simulink model "Notfalltests"  (R2021a)
settings: Solver=VariableStepAuto  StartTime=0.0  StopTime=1  RelTol=1e-3
model workspace (MAT data in the model file):
  Kz = Simulink.Parameter
  Kz.Value = Simulink.data.Expression
  Kz.Value.ExpressionString = "(L/(Lc+ds))"
  Kz.DataType = 'auto'
  Kz.Dimensions = -1
  L = Simulink.Parameter
  L.Value = 52.8
  L.DataType = 'auto'
  L.Dimensions = [1 1]
  Lc = Simulink.Parameter
  Lc.Value = 4.4
  Lc.DataType = 'auto'
  Lc.Dimensions = [1 1]
  Rk = Simulink.Parameter
  Rk.Value = Simulink.data.Expression
  Rk.Value.ExpressionString = "Lc/v"
  Rk.DataType = 'auto'
  Rk.Dimensions = -1
  Tz = Simulink.Parameter
  Tz.Value = Simulink.data.Expression
  Tz.Value.ExpressionString = "L/v"
  Tz.DataType = 'auto'
  Tz.Dimensions = -1
  ds = Simulink.Parameter
  ds.Value = Simulink.data.Expression
  ds.Value.ExpressionString = "dt*v"
  ds.DataType = 'auto'
  ds.Dimensions = -1
  dt = Simulink.Parameter
  dt.Value = 1
  dt.DataType = 'auto'
  dt.Dimensions = [1 1]
  v = Simulink.Parameter
  v.Value = 13.89
  v.DataType = 'auto'
  v.Dimensions = [1 1]
libraries: EdgesLibrary x8, StreetLanesLibrary x6, SourcesAndSinksLibrary x4, simulink x2
settings Model: OrderedModelArguments=off  Creator=phill  LastModifiedBy=phill
settings SolverCC: ZeroCrossAlgorithm=Adaptive

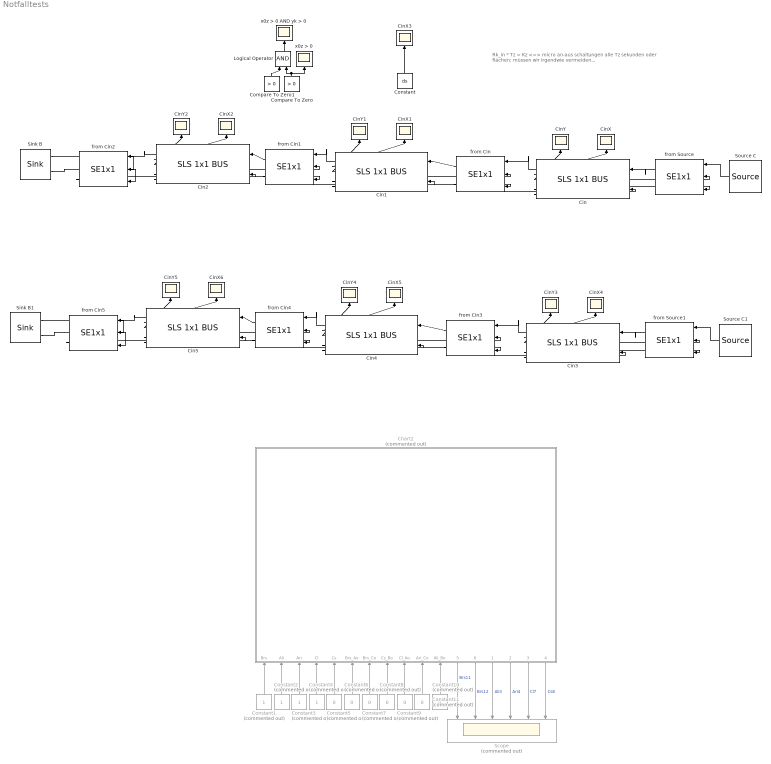
== system Notfalltests ==
  note: Rk_in * Tz = Kz   <=> micro an-aus schaltungen alle Tz sekunden
      | oder flächen; müssen wir irgendwie vermeiden...
  Chart2 : Stateflow chart  Commented=on  TreatAsAtomicUnit=on
      settings: PortSchema="{\"entries\":[{\"content\":{\"sides\":[{\"content\":{\"connectorIds\":[]},\"type\":\"ConnectorPlacement.EquallySpacedRectSide\",\"uuid\":\"dee1a780-e9dd-4205-adb9-3e9cb1ec0cd6\"},{\"content\":{\"connectorIds\":[],\"side\":\"RIGHT\"},\"type\":\"ConnectorPlacement.EquallySpacedRectSide\",\"uuid\":\"bc6af08d-2df8-4a74-93d0-032b7c1c381c\"},{\"content\":{\"connectorIds\":[],\"side\":\"TOP\"},\"type\":\"ConnectorPlacement.EquallySpacedRectSide\",\"uuid\":\"98fea325-c9fc-472d-8e1a-d846d6e99e12\"},{\"content\":{\"connectorIds\":[\"In5\",\"In1\",\"In2\",\"In3\",\"In4\",\"In11\",\"In10\",\"In9\",\"In8\",\"In7\",\"In6\",\"Out5\",\"Out6\",\"Out1\",\"Out2\",\"Out3\",\"Out4\"],\"side\":\"BOTTOM\"},\"type\":\"ConnectorPlacement.EquallySpacedRectSide\",\"uuid\":\"a092283f-ef46-48e2-a5f8-8210ac00b2f9\"}]},\"type\":\"ConnectorPlacement.EquallySpacedConnector\",\"uuid\":\"33a851aa-4180-41c0-b4bb-9b9c3be41936\"}],\"packageUris\":[\"http://schema.mathworks.com/mf0/Connector/R2020b\"],\"version\":\"1.0\"}"
  Cin : StreetLanesLibrary/SLS 1x1 BUS  Kz=2.886  Tz=3.8
  Cin1 : StreetLanesLibrary/SLS 1x1 BUS  Kz=2.886  Tz=3.8
  Cin2 : StreetLanesLibrary/SLS 1x1 BUS  Kz=2.886  Tz=3.8
  Cin3 : StreetLanesLibrary/SLS 1x1 BUS  Kz=1  Tz=1
  Cin4 : StreetLanesLibrary/SLS 1x1 BUS  Kz=1  Tz=1
  Cin5 : StreetLanesLibrary/SLS 1x1 BUS  Kz=1  Tz=1
  CinX{,1..6} (7 alike) : Scope
  CinY{,1..5} (6 alike) : Scope
  Compare To Zero : simulink/Logic and Bit Operations/Compare To Zero  relop=>  OutDataTypeStr=boolean
  Compare To Zero1 : simulink/Logic and Bit Operations/Compare To Zero  relop=>  OutDataTypeStr=boolean
  Constant : Constant  Value=ds
  Constant{1..4} (4 alike) : Constant  Commented=on
  Constant{5..11} (7 alike) : Constant  Commented=on  Value=0
  Logical Operator : Logic  AllPortsSameDT=off  OutDataTypeStr=boolean
  Scope : Scope  Commented=on  NumInputPorts=6
  Sink B : SourcesAndSinksLibrary/Sink  SystemSampleTime=-1  VariantActivationTime=update diagram  Latency=0  AutoFrameSizeCalculation=off
      settings: PortSchema="{\"entries\":[{\"content\":{\"sides\":[{\"content\":{\"connectorIds\":[\"Out1\",\"Out2\"]},\"type\":\"ConnectorPlacement.EquallySpacedRectSide\",\"uuid\":\"9fd2383e-3590-4f0f-bafc-5a4adfbb32b4\"},{\"content\":{\"connectorIds\":[],\"side\":\"RIGHT\"},\"type\":\"ConnectorPlacement.EquallySpacedRectSide\",\"uuid\":\"1e687aa9-1098-45bd-a1f6-ea403f3f2897\"},{\"content\":{\"connectorIds\":[],\"side\":\"TOP\"},\"type\":\"ConnectorPlacement.EquallySpacedRectSide\",\"uuid\":\"fe6eaa71-085c-414b-983a-a0e72e52a49c\"}]},\"type\":\"ConnectorPlacement.EquallySpacedConnector\",\"uuid\":\"370c1712-4373-4726-99c2-6cb04807ece1\"}],\"packageUris\":[\"http://schema.mathworks.com/mf0/Connector/R2020b\"],\"version\":\"1.0\"}"
  Sink B1 : SourcesAndSinksLibrary/Sink  SystemSampleTime=-1  VariantActivationTime=update diagram  Latency=0  AutoFrameSizeCalculation=off
      settings: PortSchema="{\"entries\":[{\"content\":{\"sides\":[{\"content\":{\"connectorIds\":[\"Out1\",\"Out2\"]},\"type\":\"ConnectorPlacement.EquallySpacedRectSide\",\"uuid\":\"9fd2383e-3590-4f0f-bafc-5a4adfbb32b4\"},{\"content\":{\"connectorIds\":[],\"side\":\"RIGHT\"},\"type\":\"ConnectorPlacement.EquallySpacedRectSide\",\"uuid\":\"1e687aa9-1098-45bd-a1f6-ea403f3f2897\"},{\"content\":{\"connectorIds\":[],\"side\":\"TOP\"},\"type\":\"ConnectorPlacement.EquallySpacedRectSide\",\"uuid\":\"fe6eaa71-085c-414b-983a-a0e72e52a49c\"}]},\"type\":\"ConnectorPlacement.EquallySpacedConnector\",\"uuid\":\"370c1712-4373-4726-99c2-6cb04807ece1\"}],\"packageUris\":[\"http://schema.mathworks.com/mf0/Connector/R2020b\"],\"version\":\"1.0\"}"
  Source C : SourcesAndSinksLibrary/Source  SystemSampleTime=-1  VariantActivationTime=update diagram  Latency=0  AutoFrameSizeCalculation=off
  Source C1 : SourcesAndSinksLibrary/Source  SystemSampleTime=-1  VariantActivationTime=update diagram  Latency=0  AutoFrameSizeCalculation=off
  from Cin : EdgesLibrary/SE1x1  Rk=0.32
  from Cin1 : EdgesLibrary/SE1x1  Rk=0.32
  from Cin2 : EdgesLibrary/SE1x1  Rk=0.32
  from Cin3 : EdgesLibrary/SE1x1  Rk=1
  from Cin4 : EdgesLibrary/SE1x1  Rk=1
  from Cin5 : EdgesLibrary/SE1x1  Rk=1
  from Source : EdgesLibrary/SE1x1  Rk=0.32
  from Source1 : EdgesLibrary/SE1x1  Rk=1
  x0z > 0 : Scope
  x0z > 0 AND yk > 0 : Scope
  wires:
  Cin/3 -> CinX/1
  Cin/7 -> from Source/3
  Cin/4 -> CinY/1
  Source C/1 -> from Source/1
  Cin/6 -> from Source/2
  from Source/1 -> Cin/1
  from Cin/2 -> Cin/2
  Cin/2 -> from Cin/1
  Cin1/6 -> from Cin/2
  Cin1/7 -> from Cin/3
  from Cin/1 -> Cin1/1
  Cin1/4 -> CinY1/1
  Cin1/3 -> CinX1/1
  Cin1/2 -> from Cin1/1
  from Cin1/2 -> Cin1/2
  Compare To Zero1/1 -> Logical Operator/1
  Compare To Zero/1 -> Logical Operator/2, x0z > 0/1
  Logical Operator/1 -> x0z > 0 AND yk > 0/1
  Sink B/1 -> from Cin2/2
  Sink B/2 -> from Cin2/3
  Cin2/2 -> from Cin2/1
  from Cin2/2 -> Cin2/2
  Cin2/6 -> from Cin1/2
  Cin2/7 -> from Cin1/3
  from Cin1/1 -> Cin2/1
  Cin2/4 -> CinY2/1
  Cin2/3 -> CinX2/1
  Constant/1 -> CinX3/1
  Constant11/1 -> Chart2/7(Ari_Co)
  Constant9/1 -> Chart2/8(Cl_Ao)
  Constant7/1 -> Chart2/10(Brs_Co)
  Constant3/1 -> Chart2/2(Ari)
  Constant2/1 -> Chart2/1(Ali)
  Constant8/1 -> Chart2/9(Cs_Bo)
  Constant6/1 -> Chart2/11(Brs_Ao)
  Constant1/1 -> Chart2/5(Brs)
  Chart2/6(enableBrs12) -> Scope/2  "Brs12"
  Chart2/1(enableAli3) -> Scope/3  "Ali3"
  Chart2/2(enableAri4) -> Scope/4  "Ari4"
  Constant4/1 -> Chart2/3(Cl)
  Constant10/1 -> Chart2/6(Ali_Bo)
  Chart2/3(enableCl7) -> Scope/5  "Cl7"
  Chart2/4(enableCs8) -> Scope/6  "Cs8"
  Constant5/1 -> Chart2/4(Cs)
  Chart2/5(enableBrs11) -> Scope/1  "Brs11"
  Sink B1/1 -> from Cin5/2
  from Cin4/1 -> Cin5/1
  from Source1/1 -> Cin3/1
  Cin5/7 -> from Cin4/3
  Cin3/6 -> from Source1/2
  from Cin5/2 -> Cin5/2
  Cin5/6 -> from Cin4/2
  Cin5/4 -> CinY5/1
  Cin5/3 -> CinX6/1
  Cin5/2 -> from Cin5/1
  Source C1/1 -> from Source1/1
  Cin4/2 -> from Cin4/1
  Sink B1/2 -> from Cin5/3
  Cin4/7 -> from Cin3/3
  Cin3/2 -> from Cin3/1
  from Cin3/1 -> Cin4/1
  from Cin3/2 -> Cin3/2
  Cin4/6 -> from Cin3/2
  Cin4/4 -> CinY4/1
  Cin3/7 -> from Source1/3
  from Cin4/2 -> Cin4/2
  Cin3/3 -> CinX4/1
  Cin3/4 -> CinY3/1
  Cin4/3 -> CinX5/1

== stateflow chart Notfalltests/Chart2 ==
  note: Notizen (mal auf Deutsch):
      | wenn an einer kante etwas anliegt und keine der stärkeren kanten etwas anliegen hat,
      | und die konfliktbereiche frei sind: schalte kante frei
      | <Ali 3> wird dominiert von <Cl 7> und <Cs 8> [Kreuzungen: <Brs Co> <Cl Ao> <Cs Bo>
      | <Ari 4> wird nicht dominiert [Kreuzungen: <Brs Co>
      | <Cl 7> wird dominiert von <Brs 11> und <Brs 12> [Kreuzungen: <Brs Co> <Brs Ao><Ali Bo>
      | <Cs 8> wird nicht dominiert [Kreuzungen: <Ali Bo>
      | <Brs 11> wird dominiert von <Ali 3> und <Ari 4> [Kreuzungen: <Brs Ao> <Ali Bo> <Ari Co>*<Cl Ao>
      | <Brs 12> wird nicht dominiert [Kreuzungen: <Cl Ao>
      |
      | Anmerkung: die einflüsse Brs11 und Brs12 behindern sich nicht. da beide kanten an
      | EIN UND DEMSELBEN SEGMENT liegen, und unsere 0.5:0.5 gewichtung schon suggeriert,
      | dass sich hier die autos "spalten", können sich die autos beim "Parallelen" fließen
      | in die segmente <Brs Co> und <Brs Ao> nicht wirklich in die quere kommen. Oder selbst wenn sie es
      | tun, können wir nichts dagegen unternehmen - wenn wir einem der pfade gegenüber dem anderen
      | priorität geben, wird bei dem anderen jeweils NIE etwas fließen. Damit müssen wir wohl leben :(
      |
      | a)
      | if [Ali > 0 && Cl == 0 && Cs == 0 && Brs_Co == 0 && Cl_Ao == 0 && Cs_Bo == 0]{enableAli3=1;}
      | else {enableAli3=0;}
      | b)
      | if [Ari > 0 && Brs_Co == 0]{enableAri4=1;}
      | else {enableAri4=0;}
      | c)
      | if [Cl > 0 && Brs == 0 && Brs_Co == 0 && Brs_Ao == 0 && Ali_Bo == 0]{enableCl7=1;}
      | else {enableCl7=0;}
      | d)
      | if [Cs > 0 && Ali_Bo == 0]{enableCs8=1;}
      | else {enableCs8=0;}
      | e)
      | if [Brs > 0 && Ali == 0 && Ari == 0 && Ali_Bo == 0 && Ari_Co == 0 && Cl_Ao]{enableBrs11=1;}
      | else {enableBrs11=0;}
      | f)
      | if [Brs > 0 && Cl_Ao == 0]{enableBrs12=1;}
      | else {enableBrs12=0;}
      |
      | Anmerkung: Da es im Falle [Ali > 0 && Brs > 0 && Cl > 0] einen deadlock gibt, müssen wir uns entscheiden, wer fahren darf.
      |
      | // Brs11 soll das fahrtrecht bekommen, um den fluss entlang der geraden aufrechtzuerhalten, wenn möglich
      | if [Ari == 0 && (Ali_Bo == 0 && Ari_Co == 0 && Cl_Ao == 0)]{enableBrs11=1;}
      | else
      |
      | // falls Brs12 nicht kann, versucht Ali zu fahren. Eigentlich müsste Cl die nächstbeste Wahl sein,
      | // allerdings kann Cl im falle eines Deadlocks ohnehin nicht fließen, da wegen unserer modellierung
      | // der 1x2 kanten (bzw. 1x2 segmente) gilt "Deadlock => [Brs > 0] => [Brs12 will aktiv sein]" - und da
      | // Brs12 vorrang vor Cl7 hat, ist Cl7 in diesem szenario grundsätzlich blockiert.
      | if [Cs == 0 && (Brs_Co == 0 && Cl_Ao == 0 && Cs_Bo == 0)]{enableAli3=1;}
      | else //guess noone can make it
  note: ?
  note: Brs-11-<Brs Co>-6-Co
      | (Links will geradeaus)
  note: Brs-12-<Brs Ao>-1-Ao
      | (Links will geradeaus)
  note: Ari-4-<Ari Co>-5-Co
      | (Unten will rechts abbiegen)
  note: Cl-7-<Cl Ao>-2-Ao
      | (Rechts will links abbiegen)
  note: Cs-8-<Cl Ao>-9-Bo
      | (Rechts will geradeaus)
  note: Ali-3-<Ali Bo>-10-Bo
      | (Unten will Links abbiegen)
  note: Deadlock-Detection
  note: Anstelle der ebene für deadlock resolution konnte man den "Links will geradeaus" bereich in der reihenfolge VOR "Unten will links abbiegen" setzen. "Links will geradeaus" muss dann um eine weitere kante mit höchster priorität ergänzt werden mit einem label
      | [ (Ali > 0 && Brs > 0 && Cl > 0 ) && (Ari == 0 && Ali_Bo == 0 && Ari_Co == 0]{enableBrs11=1;}
      |
      | "Unten will links abbiegen" wird dann ebenfalls um eine Kante mit höchster priorität ergänzt mit dem Label
      | [ (Ali > 0 && Brs > 0 && Cl > 0) && (Cs_Bo == 0 && Cl_Ao == 0) && ~(enableBrs11==1)
  note: Deadlock-Resolution
  (junction 23) -> (junction 29) [order 1] : [Ari > 0 && Brs_Co == 0]{enableAri4=1;}
  (junction 29) -> (junction 36) [order 1] : [Cl > 0 && Brs == 0 && Brs_Co == 0 && Brs_Ao == 0 && Ali_Bo == 0]{enableCl7=1; }
  (junction 39) -> (junction 40) [order 1] : [Brs > 0 && Ali == 0 && Ari == 0 && Ali_Bo == 0 && Ari_Co == 0 && Cl_Ao]{enableBrs11=1;}
  (junction 40) -> (junction 45) [order 1] : [Brs > 0 && Cl_Ao == 0]{enableBrs12=1;}
  (junction 36) -> (junction 39) [order 1] : [Cs > 0 && Ali_Bo == 0]{enableCs8=1;}
  (junction 79) -> (junction 23) [order 1] : [Ali > 0 && Cl == 0 && Cs == 0 && Brs_Co == 0 && Cl_Ao == 0 && Cs_Bo == 0]
      | {enableAli3=1; }
  (junction 39) -> (junction 40) [order 2] : {enableBrs11=0;}
  (junction 79) -> (junction 23) [order 2] : {enableAli3=0;}
  (junction 29) -> (junction 36) [order 2] : {enableCl7=0;}
  (junction 36) -> (junction 39) [order 2] : {enableCs8=0;}
  (junction 23) -> (junction 29) [order 2] : {enableAri4=0;}
  (junction 40) -> (junction 45) [order 2] : {enableBrs12=0;}
  (junction 45) -> (junction 53)
  (default) -> (junction 79) : {enableAli3 = 0; enableAri4 = 0;
      | enableCl7 = 0; enableCs8 = 0;
      | enableBrs11 = 0; enableBrs12 = 0;}
  (junction 53) -> (junction 80) [order 2]
  (junction 53) -> (junction 64) [order 1] : [Ali > 0 && Brs > 0 && Cl > 0]
  (junction 71) -> (junction 80)
  (junction 64) -> (junction 71) [order 1] : [Ari == 0 && (Ali_Bo == 0 && Ari_Co == 0 && Cl_Ao == 0)]{enableBrs11=1;}
  (junction 64) -> (junction 71) [order 2] : [Ari > 0 && Cs == 0 && (Brs_Co == 0 && Cl_Ao == 0 && Cs_Bo == 0)]{enableAli3=1;}
  data: Ali input; Ari input; Cl input; Cs input; Brs input; Ali_Bo input; Ari_Co input; Cl_Ao input; Cs_Bo input; Brs_Co input; Brs_Ao input; enableAli3 output; enableAri4 output; enableCl7 output; enableCs8 output; enableBrs11 output; enableBrs12 output
